simulink model "NetworkModelIntermediateIntersectionCRCA"  (R2018b)
settings: Solver=VariableStepAuto  StartTime=0.0  StopTime=10.0  RelTol=1e-3
values from neighbouring files (symbols this model uses):
  Ax = [0 1  0   0 ... (first row only)    [DroneSubsystemModelling.m]
  Ay = [0 1  0   0 ... (first row only)    [DroneSubsystemModelling.m]
  Bx = [0;0;0;b1]    [DroneSubsystemModelling.m]
  By = [0;0;0;b2]    [DroneSubsystemModelling.m]
  ConflictDrone1andDrone2 = ControlDetectionFunction(tout,PositionXDrone1TEST, PositionYDrone1TEST, PositionXDrone2TEST, PositionYDrone2TEST, ConflictDrone1andDrone2)    [ConflictDetectionTEST.m]
  ConflictDrone1andDrone3 = ControlDetectionFunction(tout,PositionXDrone1TEST, PositionYDrone1TEST, PositionXDrone3TEST, PositionYDrone3TEST, ConflictDrone1andDrone3)    [ConflictDetectionTEST.m]
  ConflictDrone1andDrone4 = ControlDetectionFunction(tout,PositionXDrone1TEST, PositionYDrone1TEST, PositionXDrone4TEST, PositionYDrone4TEST, ConflictDrone1andDrone4)    [ConflictDetectionTEST.m]
  ConflictDrone2andDrone3 = ControlDetectionFunction(tout,PositionXDrone2TEST, PositionYDrone2TEST, PositionXDrone3TEST, PositionYDrone3TEST, ConflictDrone2andDrone3)    [ConflictDetectionTEST.m]
  ConflictDrone2andDrone4 = ControlDetectionFunction(tout,PositionXDrone2, PositionYDrone2, PositionXDrone4, PositionYDrone4, ConflictDrone2andDrone4)    [ConflictDetection.m]    (also in ConflictDetectionTEST.m = ControlDetectionFunction(tout,PositionXDrone2TEST, PositionY)
  ConflictDrone3andDrone4 = ControlDetectionFunction(tout,PositionXDrone3TEST, PositionYDrone3TEST, PositionXDrone4TEST, PositionYDrone4TEST, ConflictDrone3andDrone4)    [ConflictDetectionTEST.m]
  ConflictDrone7andDrone8 = ControlDetectionFunction(tout,PositionXDrone7TEST, PositionYDrone7TEST, PositionXDrone8TEST, PositionYDrone8TEST, ConflictDrone7andDrone8)    [ConflictDetectionTEST.m]
  Cpx = [1 0 0 0]    [DroneSubsystemModelling.m]
  Cpy = [1 0 0 0]    [DroneSubsystemModelling.m]
  Cvx = [0 1 0 0]    [DroneSubsystemModelling.m]
  Cvy = [0 1 0 0]    [DroneSubsystemModelling.m]
  theta1 = -180    [MotionModelling.m]
  theta2 = -3*180/4    (= -135)    [MotionModelling.m]
  theta3 = -2*180/4    (= -90)    [MotionModelling.m]
  theta4 = -180/4    (= -45)    [MotionModelling.m]
  theta5 = 2*180    (= 360)    [MotionModelling.m]
  theta6 = 180/4    (= 45)    [MotionModelling.m]
  theta7 = 2*180/4    (= 90)    [MotionModelling.m]
  theta8 = 3*180/4    (= 135)    [MotionModelling.m]
  VelocityStarX1 = vx10    [MotionModelling.m]
  VelocityStarX2 = vx20    [MotionModelling.m]
  VelocityStarX3 = vx30    [MotionModelling.m]
  VelocityStarX4 = vx40    [MotionModelling.m]
  VelocityStarX5 = vx50    [MotionModelling.m]
  VelocityStarX6 = vx60    [MotionModelling.m]
  VelocityStarX7 = vx70    [MotionModelling.m]
  VelocityStarX8 = vx80    [MotionModelling.m]
  VelocityStarY1 = vy10    [MotionModelling.m]
  VelocityStarY2 = vy20    [MotionModelling.m]
  VelocityStarY3 = vy30    [MotionModelling.m]
  VelocityStarY4 = vy40    [MotionModelling.m]
  VelocityStarY5 = vy50    [MotionModelling.m]
  VelocityStarY6 = vy60    [MotionModelling.m]
  VelocityStarY7 = vy70    [MotionModelling.m]
  VelocityStarY8 = vy80    [MotionModelling.m]
  X10 = [x10 vx10 0 0]'    [MotionModelling.m]
  X20 = [x20 vx20 0 0]'    [MotionModelling.m]
  X30 = [x30 vx30 0 0]'    [MotionModelling.m]
  X40 = [x40 vx40 0 0]'    [MotionModelling.m]
  X50 = [x50 vx50 0 0]'    [MotionModelling.m]
  X60 = [x60 vx60 0 0]'    [MotionModelling.m]
  X70 = [x70 vx70 0 0]'    [MotionModelling.m]
  X80 = [x80 vx80 0 0]'    [MotionModelling.m]
  Y10 = [y10 vy10 0 0]'    [MotionModelling.m]
  Y20 = [y20 vy20 0 0]'    [MotionModelling.m]
  Y30 = [y30 vy30 0 0]'    [MotionModelling.m]
  Y40 = [y40 vy40 0 0]'    [MotionModelling.m]
  Y50 = [y50 vy50 0 0]'    [MotionModelling.m]
  Y60 = [y60 vy60 0 0]'    [MotionModelling.m]
  Y70 = [y70 vy70 0 0]'    [MotionModelling.m]
  Y80 = [y80 vy80 0 0]'    [MotionModelling.m]
undefined symbols (not defined in the file or in its folder): ConflictDrone5andDrone6, K
libraries: simulink x16
(part 2 of 2)

== matlab function NetworkModelIntermediateIntersectionCRCA/MATLAB Function2 ==
  data: qxA input; Vdiff output; qxB input; qxC input; qxD input; qyA input; qyB input; qyC input; qyD input; qDotxA input; qDotxB input; qDotxC input; qDotxD input; qDotyA input; qDotyB input; qDotyC input; qDotyD input; M output; N output; RANGE output; minimumClosureTime output; numOfCollisions output
function [Vdiff,M,N,RANGE,minimumClosureTime, numOfCollisions] = SpeedController(qxA,qxB,qxC,qxD, qyA, qyB, qyC, qyD, qDotxA,qDotxB,qDotxC,qDotxD, qDotyA, qDotyB, qDotyC, qDotyD)

coder.extrinsic('warning');
coder.extrinsic('wrapToPi');
coder.extrinsic('speeddifference') 

qx = [qxA, qxB,qxC,qxD];
qy = [qyA, qyB, qyC, qyD];

qDotx = [qDotxA,qDotxB,qDotxC,qDotxD];
qDoty = [qDotyA,qDotyB,qDotyC,qDotyD];

Vmax = 0.2;

%Vdiff = speeddifference(qx, qy, qDotx, qDoty);

K = 1; 
nT = length(qx);
PriorityMatrix = zeros(5,6);

collisionNumber = 0;

    for m = 1:nT

       for n = 1:nT
           
           if n>m
                          
                qxi = qx(m);
                qyi = qy(m);
                qxj = qx(n);
                qyj = qy(n);

                Range = K*sqrt((qxi - qxj)^2 + (qyi - qyj)^2); 

                qDotxi = qDotx(m);
                qDotyi = qDoty(m);
                qDotxj = qDotx(n);
                qDotyj = qDoty(n);

                ClosureRate = K*sqrt((qDotxi - qDotxj)^2 + (qDotyi - qDotyj)^2); 

                ClosureTime =  Range/ClosureRate;

                collisionNumber = collisionNumber + 1;
                
                Collision = [m;n;Range;ClosureRate;ClosureTime];

                PriorityMatrix(:,collisionNumber) = Collision;

           end 

       end 

    end
 




    ClosureTimeVector = PriorityMatrix(5,:);
    
    [minimumClosureTime, I] = min(ClosureTimeVector);
    
Vdiff = PriorityMatrix(4,I);
M = PriorityMatrix(1,I);
N = PriorityMatrix(2,I);
RANGE = PriorityMatrix(3,I);
numOfCollisions = collisionNumber;

%     if abs(Vdiff) >= Vmax/2
%         Vdiff = Vmax/2;
%     end 

end 

% 
% if (M-N) < nT
%     if M > N
%         if (M == 1)
%             VdiffA = -Vdiff;
%         elseif (M == 2)
%             VdiffB = -Vdiff;    
%         elseif (M == 3)
%             VdiffC = -Vdiff;    
%         elseif (M == 4)
%             VdiffD = -Vdiff;
%         end
%         
%     else
%

== matlab function NetworkModelIntermediateIntersectionCRCA/MATLAB Function3 ==
  data: qDotxi input; y output; qDotxj input; qDotyi input; qDotyj input
function y = ClosureRate(qDotxi, qDotxj, qDotyi, qDotyj)

Vmax = 0.2;
K = 1;
Vdiff = K*sqrt((qDotxi - qDotxj)^2 + (qDotyi - qDotyj)^2); 

if abs(Vdiff)>=Vmax/2
    Vdiff = Vmax/2;
end 

y = Vdiff;
